simulink model "Laplace"  (R2018a)
settings: Solver=VariableStepAuto  StartTime=0.0  StopTime=10.0  RelTol=1e-3
values from neighbouring files (symbols this model uses):
  a = 1    [Prj_4_laplace.m]
  b = 0.1    [Prj_4_laplace.m]
  c = 10    [Prj_4_laplace.m]
  F = 10    [Prj_4_laplace.m]
libraries: dspsrcs4 x1
settings Model: Creator=Admin  LastModifiedBy=Admin

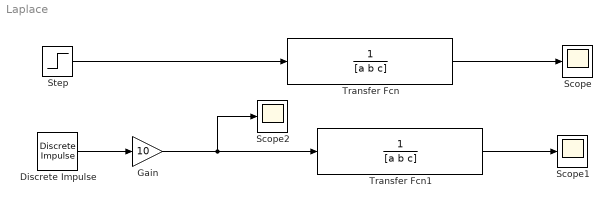
== system Laplace ==
  Discrete Impulse : dspsrcs4/Discrete  Impulse  Delay=0  SampleTime=1  FrameSample=1  OutputFrames=off  dataType=double  isSigned=on  wordLen=16  udDataType=sfix(16)  fracBitsMode=Best precision  numFracBits=15  OutDataTypeStr=double  LastOutDataTypeStr=double
  Gain : Gain  Gain=10
  Scope : Scope
  Scope1 : Scope
  Scope2 : Scope
  Step : Step  Time=0  After=F  SampleTime=0.1
  Transfer Fcn : TransferFcn  Denominator=[a b c]
  Transfer Fcn1 : TransferFcn  Denominator=[a b c]
  wires:
  Transfer Fcn/1 -> Scope/1
  Transfer Fcn1/1 -> Scope1/1
  Step/1 -> Transfer Fcn/1
  Discrete Impulse/1 -> Gain/1
  Gain/1 -> Transfer Fcn1/1, Scope2/1
